simulink library "ADDAlib"  (R2012b)
settings: Solver=ode45  StartTime=0.0  StopTime=10.0  RelTol=1e-3
settings Model: Creator=nian  LastModifiedBy=nian

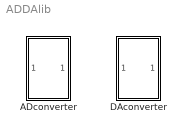
== system ADDAlib ==
  ADconverter : Subsystem  mask{Vinmin=-10, Vinmax=9.995, ADoutmin=0, ADoutmax=4095, Tsample=0.01}
      mask prompts: Vinmin "Vin min"; Vinmax "Vin max"; ADoutmin "ADout min"; ADoutmax "ADout max"; Tsample "Sampletime"
  DAconverter : Subsystem  mask{Voutmin=-10, Voutmax=9.995, DAinmin=0, DAinmax=4095, Tsample=0.01}
      mask prompts: Voutmin "Vout min"; Voutmax "Vout max"; DAinmin "DAin min"; DAinmax "DAin max"; Tsample "Sampletime"

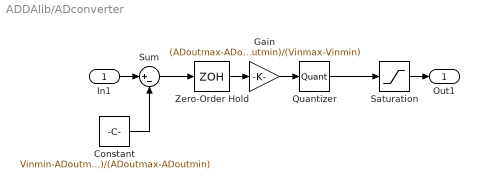
== system ADDAlib/ADconverter ==
  In1 : Inport
  Constant : Constant  Value=Vinmin-ADoutmin*(Vinmax-Vinmin)/(ADoutmax-ADoutmin)
  Gain : Gain  Gain=(ADoutmax-ADoutmin)/(Vinmax-Vinmin)
  Quantizer : Quantizer  QuantizationInterval=1
  Saturation : Saturate  UpperLimit=ADoutmax  LowerLimit=ADoutmin
  Sum : Sum  Inputs=|+-
  Zero-Order Hold : ZeroOrderHold  SampleTime=Tsample
  Out1 : Outport
  wires:
  Quantizer/1 -> Saturation/1
  Constant/1 -> Sum/2
  Gain/1 -> Quantizer/1
  In1/1 -> Sum/1
  Saturation/1 -> Out1/1
  Zero-Order Hold/1 -> Gain/1
  Sum/1 -> Zero-Order Hold/1

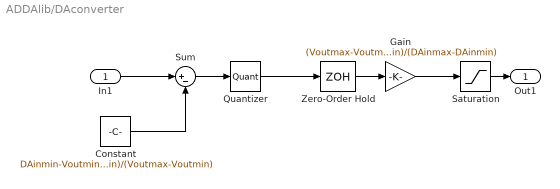
== system ADDAlib/DAconverter ==
  In1 : Inport
  Constant : Constant  Value=DAinmin-Voutmin*(DAinmax-DAinmin)/(Voutmax-Voutmin)
  Gain : Gain  Gain=(Voutmax-Voutmin)/(DAinmax-DAinmin)
  Quantizer : Quantizer  QuantizationInterval=1
  Saturation : Saturate  UpperLimit=Voutmax  LowerLimit=Voutmin
  Sum : Sum  Inputs=|+-
  Zero-Order Hold : ZeroOrderHold  SampleTime=Tsample
  Out1 : Outport
  wires:
  Constant/1 -> Sum/2
  In1/1 -> Sum/1
  Saturation/1 -> Out1/1
  Zero-Order Hold/1 -> Gain/1
  Gain/1 -> Saturation/1
  Quantizer/1 -> Zero-Order Hold/1
  Sum/1 -> Quantizer/1
